simulink model "Sim_MEMSFixed_CS2"  (R2021b)
settings: Solver=VariableStepAuto  StartTime=0.0  StopTime=10  MaxStep=0.001  RelTol=1e-3
settings Model: Creator=Rasoul  LastModifiedBy=Rasoul

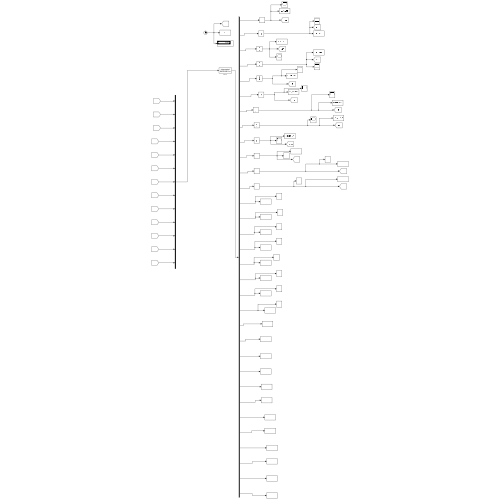
[thumbnail: Simulink's stored preview of the top-level diagram]
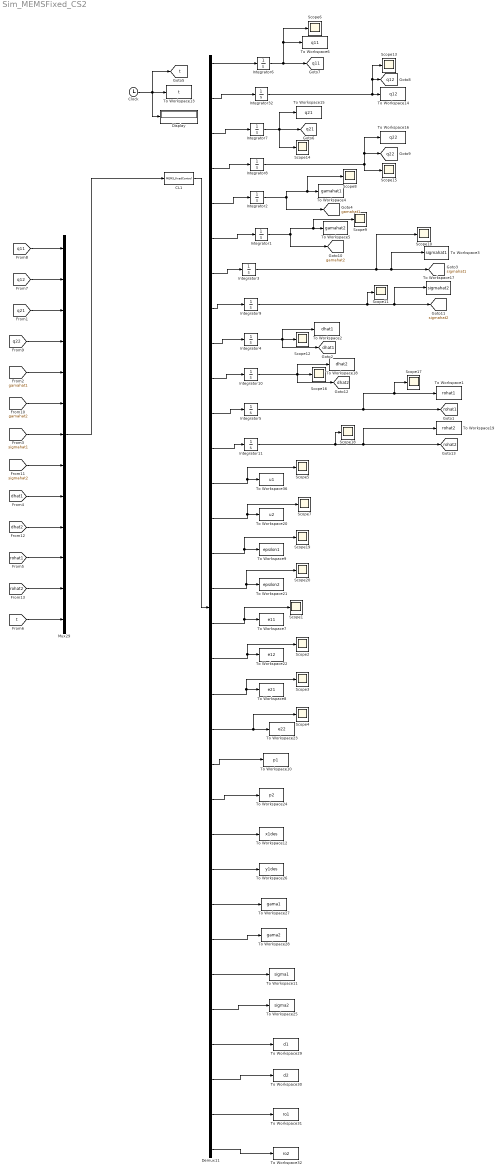
== system Sim_MEMSFixed_CS2 ==
  CL1 : MATLABFcn  MATLABFcn=MEMS_fixedControl  OutputDimensions=32  Output1D=off
  Clock : Clock
      settings: Decimation=1000
  Demux11 : Demux  Outputs=32
  Display : Display
      settings: Decimation=1000
  Integrator1 : Integrator  InitialCondition=-2
  Integrator10 : Integrator  InitialCondition=0.75
  Integrator11 : Integrator  InitialCondition=1
  Integrator2 : Integrator  InitialCondition=-2
  Integrator3 : Integrator  InitialCondition=-1.25
  Integrator32 : Integrator  InitialCondition=-0.38
  Integrator4 : Integrator  InitialCondition=0.6
  Integrator5 : Integrator  InitialCondition=1
  Integrator6 : Integrator  InitialCondition=-0.73
  Integrator7 : Integrator
  Integrator8 : Integrator
  Integrator9 : Integrator  InitialCondition=-1.25
  Mux29 : Mux  Inputs=13
  Scope{1..20} (20 alike) : Scope
  To Workspace1 : ToWorkspace  VariableName=rohat1  SampleTime=0.001
      settings: Save2DSignal=2-D array (concatenate along first dimension)
  To Workspace10 : ToWorkspace  VariableName=p1  SampleTime=0.001
      settings: Save2DSignal=2-D array (concatenate along first dimension)
  To Workspace11 : ToWorkspace  VariableName=sigma1  SampleTime=0.001
      settings: Save2DSignal=2-D array (concatenate along first dimension)
  To Workspace12 : ToWorkspace  VariableName=x1des  SampleTime=0.001
      settings: Save2DSignal=2-D array (concatenate along first dimension)
  To Workspace13 : ToWorkspace  VariableName=t  SampleTime=0.001
      settings: Save2DSignal=2-D array (concatenate along first dimension)
  To Workspace14 : ToWorkspace  VariableName=q12  SampleTime=0.001
      settings: Save2DSignal=2-D array (concatenate along first dimension)
  To Workspace15 : ToWorkspace  VariableName=q21  SampleTime=0.001
      settings: Save2DSignal=2-D array (concatenate along first dimension)
  To Workspace16 : ToWorkspace  VariableName=q22  SampleTime=0.001
      settings: Save2DSignal=2-D array (concatenate along first dimension)
  To Workspace17 : ToWorkspace  VariableName=sigmahat2  SampleTime=0.001
      settings: Save2DSignal=2-D array (concatenate along first dimension)
  To Workspace18 : ToWorkspace  VariableName=dhat2  SampleTime=0.001
      settings: Save2DSignal=2-D array (concatenate along first dimension)
  To Workspace19 : ToWorkspace  VariableName=rohat2  SampleTime=0.001
      settings: Save2DSignal=2-D array (concatenate along first dimension)
  To Workspace2 : ToWorkspace  VariableName=dhat1  SampleTime=0.001
      settings: Save2DSignal=2-D array (concatenate along first dimension)
  To Workspace20 : ToWorkspace  VariableName=u2  SampleTime=0.001
      settings: Save2DSignal=2-D array (concatenate along first dimension)
  To Workspace21 : ToWorkspace  VariableName=epsilon2  SampleTime=0.001
      settings: Save2DSignal=2-D array (concatenate along first dimension)
  To Workspace22 : ToWorkspace  VariableName=e12  SampleTime=0.001
      settings: Save2DSignal=2-D array (concatenate along first dimension)
  To Workspace23 : ToWorkspace  VariableName=e22  SampleTime=0.001
      settings: Save2DSignal=2-D array (concatenate along first dimension)
  To Workspace24 : ToWorkspace  VariableName=p2  SampleTime=0.001
      settings: Save2DSignal=2-D array (concatenate along first dimension)
  To Workspace25 : ToWorkspace  VariableName=sigma2  SampleTime=0.001
      settings: Save2DSignal=2-D array (concatenate along first dimension)
  To Workspace26 : ToWorkspace  VariableName=y1des  SampleTime=0.001
      settings: Save2DSignal=2-D array (concatenate along first dimension)
  To Workspace27 : ToWorkspace  VariableName=gama1  SampleTime=0.001
      settings: Save2DSignal=2-D array (concatenate along first dimension)
  To Workspace28 : ToWorkspace  VariableName=gama2  SampleTime=0.001
      settings: Save2DSignal=2-D array (concatenate along first dimension)
  To Workspace29 : ToWorkspace  VariableName=d1  SampleTime=0.001
      settings: Save2DSignal=2-D array (concatenate along first dimension)
  To Workspace3 : ToWorkspace  VariableName=sigmahat1  SampleTime=0.001
      settings: Save2DSignal=2-D array (concatenate along first dimension)
  To Workspace30 : ToWorkspace  VariableName=d2  SampleTime=0.001
      settings: Save2DSignal=2-D array (concatenate along first dimension)
  To Workspace31 : ToWorkspace  VariableName=ro1  SampleTime=0.001
      settings: Save2DSignal=2-D array (concatenate along first dimension)
  To Workspace32 : ToWorkspace  VariableName=ro2  SampleTime=0.001
      settings: Save2DSignal=2-D array (concatenate along first dimension)
  To Workspace36 : ToWorkspace  VariableName=u1  SampleTime=0.001
      settings: Save2DSignal=2-D array (concatenate along first dimension)
  To Workspace4 : ToWorkspace  VariableName=gamahat1  SampleTime=0.001
      settings: Save2DSignal=2-D array (concatenate along first dimension)
  To Workspace5 : ToWorkspace  VariableName=gamahat2  SampleTime=0.001
      settings: Save2DSignal=2-D array (concatenate along first dimension)
  To Workspace6 : ToWorkspace  VariableName=q11  SampleTime=0.001
      settings: Save2DSignal=2-D array (concatenate along first dimension)
  To Workspace7 : ToWorkspace  VariableName=e11  SampleTime=0.001
      settings: Save2DSignal=2-D array (concatenate along first dimension)
  To Workspace8 : ToWorkspace  VariableName=e21  SampleTime=0.001
      settings: Save2DSignal=2-D array (concatenate along first dimension)
  To Workspace9 : ToWorkspace  VariableName=epsilon1  SampleTime=0.001
      settings: Save2DSignal=2-D array (concatenate along first dimension)
  tag scope: dhat1=global, dhat2=global, gamahat1=global, gamahat2=global, q11=global, q12=global, q21=global, q22=global, rohat1=global, rohat2=global, sigmahat1=global, sigmahat2=global, t=global
  wires:
  Clock/1 -> To Workspace13/1, [t], Display/1
  Mux29/1 -> CL1/1
  CL1/1 -> Demux11/1
  [q11] -> Mux29/1
  Integrator3/1 -> Scope10/1, To Workspace3/1, [sigmahat1]
  Integrator2/1 -> Scope8/1, To Workspace4/1, [gamahat1]
  Demux11/2 -> Integrator32/1
  Demux11/1 -> Integrator6/1
  Demux11/13 -> Scope5/1, To Workspace36/1
  Demux11/15 -> Scope19/1, To Workspace9/1
  Demux11/19 -> Scope3/1, To Workspace8/1
  Demux11/21 -> To Workspace10/1
  [t] -> Mux29/13
  [q12] -> Mux29/2
  [q21] -> Mux29/3
  [q22] -> Mux29/4
  [gamahat1] -> Mux29/5
  [gamahat2] -> Mux29/6
  [sigmahat1] -> Mux29/7
  [sigmahat2] -> Mux29/8
  [rohat2] -> Mux29/12
  [rohat1] -> Mux29/11
  [dhat2] -> Mux29/10
  [dhat1] -> Mux29/9
  Integrator32/1 -> Scope13/1, [q12], To Workspace14/1
  Integrator6/1 -> To Workspace6/1, Scope6/1, [q11]
  Demux11/3 -> Integrator7/1
  Integrator7/1 -> Scope14/1, To Workspace15/1, [q21]
  Demux11/4 -> Integrator8/1
  Integrator8/1 -> [q22], To Workspace16/1, Scope15/1
  Demux11/5 -> Integrator2/1
  Demux11/6 -> Integrator1/1
  Integrator1/1 -> [gamahat2], Scope9/1, To Workspace5/1
  Demux11/7 -> Integrator3/1
  Integrator9/1 -> Scope11/1, [sigmahat2], To Workspace17/1
  Demux11/8 -> Integrator9/1
  Demux11/9 -> Integrator4/1
  Demux11/10 -> Integrator10/1
  Integrator10/1 -> Scope16/1, [dhat2], To Workspace18/1
  Demux11/11 -> Integrator5/1
  Integrator11/1 -> Scope18/1, To Workspace19/1, [rohat2]
  Demux11/12 -> Integrator11/1
  Demux11/14 -> Scope7/1, To Workspace20/1
  Demux11/16 -> Scope20/1, To Workspace21/1
  Demux11/17 -> Scope1/1, To Workspace7/1
  Demux11/18 -> Scope2/1, To Workspace22/1
  Demux11/20 -> Scope4/1, To Workspace23/1
  Demux11/22 -> To Workspace24/1
  Integrator4/1 -> Scope12/1, To Workspace2/1, [dhat1]
  Integrator5/1 -> [rohat1], Scope17/1, To Workspace1/1
  Demux11/23 -> To Workspace12/1
  Demux11/24 -> To Workspace26/1
  Demux11/25 -> To Workspace27/1
  Demux11/26 -> To Workspace28/1
  Demux11/28 -> To Workspace25/1
  Demux11/27 -> To Workspace11/1
  Demux11/29 -> To Workspace29/1
  Demux11/30 -> To Workspace30/1
  Demux11/31 -> To Workspace31/1
  Demux11/32 -> To Workspace32/1
